simulink model "pid_test_smith"  (Simulink 6.1)
settings: Solver=ode3  StartTime=0.0  StopTime=40  FixedStep=0.01  RelTol=1e-3
libraries: simulink x1
settings Model: LastModifiedBy=murahasi
settings DebuggingCC: SolverPrmCheckMsg=warning

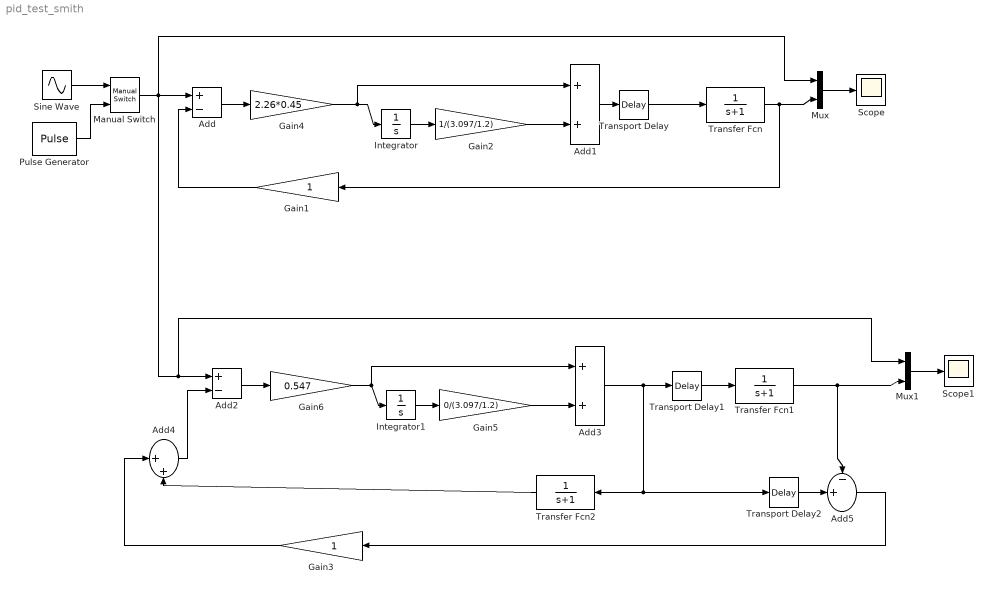
== system pid_test_smith ==
  Add : Sum  Inputs=+-  OutScaling=2^-10
  Add1 : Sum  OutScaling=2^-10
  Add2 : Sum  Inputs=+-  OutScaling=2^-10
  Add3 : Sum  OutScaling=2^-10
  Add4 : Sum  Inputs=|++  OutScaling=2^-10
  Add5 : Sum  Inputs=-+|  OutScaling=2^-10
  Gain1 : Gain  Orientation=left
  Gain2 : Gain  Gain=1/(3.097/1.2)
  Gain3 : Gain  Orientation=left
  Gain4 : Gain  Gain=2.26*0.45
  Gain5 : Gain  Gain=0/(3.097/1.2)
  Gain6 : Gain  Gain=0.547
  Integrator : Integrator
  Integrator1 : Integrator
  Manual Switch : simulink/Signal Routing/Manual Switch  sw=0  action=0
  Mux : Mux  Inputs=2
  Mux1 : Mux  Inputs=2
  Pulse Generator : DiscretePulseGenerator  PulseType=Time based  Period=30  PulseWidth=50
  Scope : Scope
  Scope1 : Scope
  Sine Wave : Sin  Frequency=2*pi*1  SampleTime=0
  Transfer Fcn : TransferFcn  Denominator=[1 1]
  Transfer Fcn1 : TransferFcn  Denominator=[1 1]
  Transfer Fcn2 : TransferFcn  Orientation=left  Denominator=[1 1]
  Transport Delay : TransportDelay
  Transport Delay1 : TransportDelay
  Transport Delay2 : TransportDelay
  wires:
  Add1/1 -> Transport Delay/1
  Add/1 -> Gain4/1
  Manual Switch/1 -> Add/1, Mux/1, Mux1/1, Add2/1
  Transfer Fcn/1 -> Mux/2, Gain1/1
  Mux/1 -> Scope/1
  Sine Wave/1 -> Manual Switch/1
  Pulse Generator/1 -> Manual Switch/2
  Integrator/1 -> Gain2/1
  Gain2/1 -> Add1/2
  Gain4/1 -> Add1/1, Integrator/1
  Gain1/1 -> Add/2
  Transport Delay/1 -> Transfer Fcn/1
  Add3/1 -> Transport Delay1/1, Transfer Fcn2/1, Transport Delay2/1
  Add2/1 -> Gain6/1
  Transfer Fcn1/1 -> Add5/1, Mux1/2
  Mux1/1 -> Scope1/1
  Integrator1/1 -> Gain5/1
  Gain5/1 -> Add3/2
  Gain6/1 -> Add3/1, Integrator1/1
  Transport Delay1/1 -> Transfer Fcn1/1
  Add4/1 -> Add2/2
  Gain3/1 -> Add4/1
  Transfer Fcn2/1 -> Add4/2
  Transport Delay2/1 -> Add5/2
  Add5/1 -> Gain3/1
